simulink model "experiment9"  (R2020b)
settings: Solver=VariableStepAuto  StartTime=0.0  StopTime=10.0  RelTol=1e-3
settings Model: Creator=LENOVO  LastModifiedBy=LENOVO

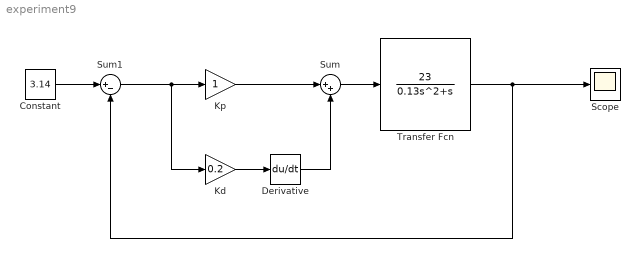
== system experiment9 ==
  Constant : Constant  Value=3.14
  Derivative : Derivative
  Kd : Gain  Gain=0.2
  Kp : Gain
  Scope : Scope
  Sum : Sum  Inputs=|++
  Sum1 : Sum  Inputs=|+-
  Transfer Fcn : TransferFcn  Numerator=[23]  Denominator=[0.13 1 0]
  wires:
  Sum/1 -> Transfer Fcn/1
  Derivative/1 -> Sum/2
  Kd/1 -> Derivative/1
  Kp/1 -> Sum/1
  Sum1/1 -> Kd/1, Kp/1
  Constant/1 -> Sum1/1
  Transfer Fcn/1 -> Sum1/2, Scope/1
